simulink model "MRAC"  (R2022a)
settings: Solver=FixedStepAuto  StartTime=0.0  StopTime=25.0  FixedStep=0.0001  RelTol=1e-3
libraries: cstblocks x5
settings Model: Creator=loryb  LastModifiedBy=loryb

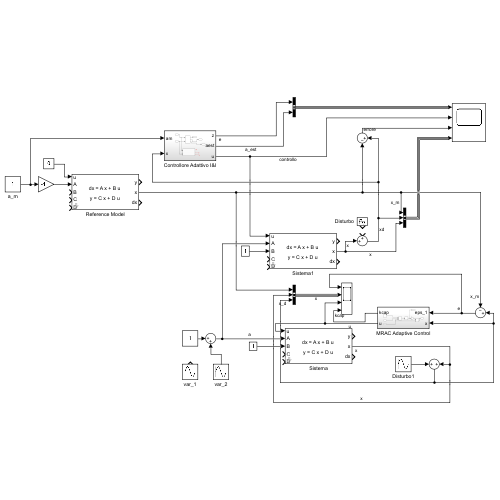
[thumbnail: Simulink's stored preview of the top-level diagram]
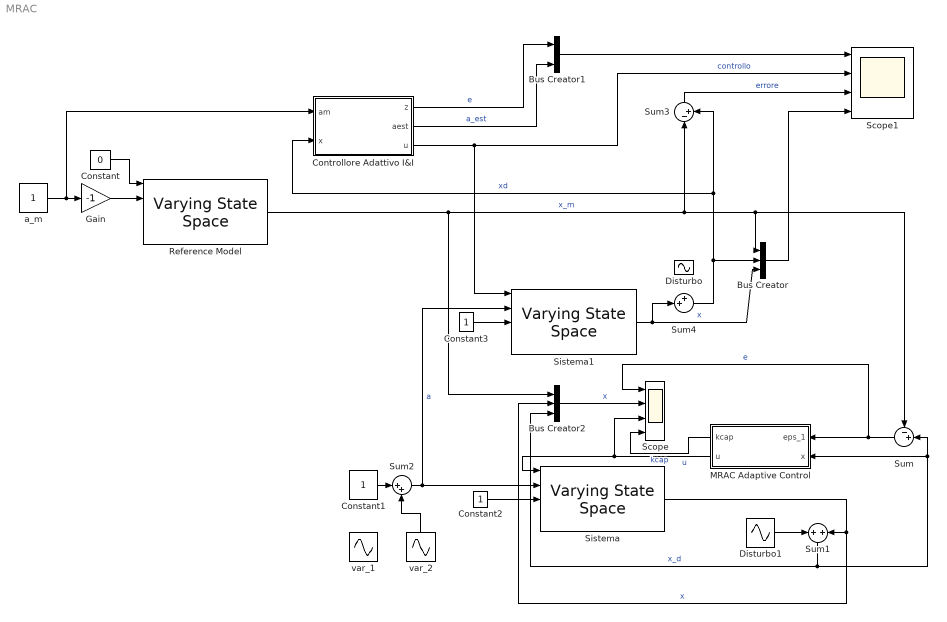
== system MRAC ==
  Bus Creator : BusCreator  Inputs=3
  Bus Creator1 : BusCreator  Inputs=2
  Bus Creator2 : BusCreator  Inputs=3
  Constant : Constant  Value=0
  Constant1 : Constant
  Constant2 : Constant
  Constant3 : Constant
  Controllore Adattivo I&I : Subsystem
  Disturbo : Sin  Amplitude=0.1  Frequency=1/5  SampleTime=0
  Disturbo1 : Sin  Amplitude=0.1  Frequency=1/5  SampleTime=0
  Gain : Gain  Gain=-1
  MRAC Adaptive Control : Subsystem
  Reference Model : cstblocks/Linear Parameter Varying/Varying State Space  x0=1  xNames=''  OutputX=on  OutputDX=on
  Scope : Scope  NumInputPorts=4
  Scope1 : Scope  NumInputPorts=4
  Sistema : cstblocks/Linear Parameter Varying/Varying State Space  x0=1  xNames=''  OutputX=on  OutputDX=on
  Sistema1 : cstblocks/Linear Parameter Varying/Varying State Space  x0=1  xNames=''  OutputX=on  OutputDX=on
  Sum : Sum  Inputs=-+|
  Sum1 : Sum  Inputs=+|+
  Sum2 : Sum  Inputs=|++
  Sum3 : Sum  Inputs=|-+
  Sum4 : Sum  Inputs=++|
  a_m : Constant
  var_1 : Sin  Amplitude=1/10  Frequency=10  SampleTime=0
  var_2 : Sin  Amplitude=10  Frequency=1/10  SampleTime=0
  wires:
  Constant/1 -> Reference Model/1
  Sum3/1 -> Scope1/3  "errore"
  Bus Creator/1 -> Scope1/4
  Controllore Adattivo I&I/1(z) -> Bus Creator1/1  "e"
  Sistema/2 -> Bus Creator2/2, Sum1/2  "x"
  Constant1/1 -> Sum2/1
  Constant3/1 -> Sistema1/3
  Bus Creator1/1 -> Scope1/1
  MRAC Adaptive Control/1(kcap) -> Scope/4  "kcap"
  Bus Creator2/1 -> Scope/2  "x"
  Constant2/1 -> Sistema/3
  Sum4/1 -> Bus Creator/2, Sum3/2, Controllore Adattivo I&I/2(x)  "xd"
  Sistema1/2 -> Bus Creator/3, Sum4/2  "x"
  Controllore Adattivo I&I/3(u) -> Scope1/2, Sistema1/1  "controllo"
  Sum2/1 -> Sistema1/2, Sistema/2  "a"
  Sum1/1 -> Bus Creator2/3, MRAC Adaptive Control/2(x), Sum/2  "x_d"
  MRAC Adaptive Control/2(u) -> Scope/3, Sistema/1  "u"
  Sum/1 -> Scope/1, MRAC Adaptive Control/1(eps_1)  "e"
  a_m/1 -> Gain/1, Controllore Adattivo I&I/1(am)
  Reference Model/2 -> Bus Creator/1, Sum/1, Sum3/1, Bus Creator2/1  "x_m"
  Controllore Adattivo I&I/2(aest) -> Bus Creator1/2  "a_est"
  Gain/1 -> Reference Model/2
  Disturbo1/1 -> Sum1/1
  var_2/1 -> Sum2/2

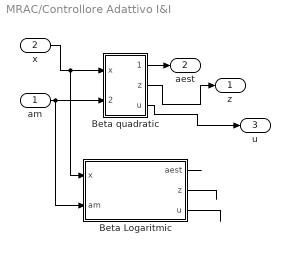
== system MRAC/Controllore Adattivo I&I ==
  am : Inport
  x : Inport  Port=2
  Beta Logaritmic : Subsystem
  Beta quadratic : Subsystem
  z : Outport
  aest : Outport  Port=2
  u : Outport  Port=3
  wires:
  x/1 -> Beta Logaritmic/1(x), Beta quadratic/1(x)
  am/1 -> Beta Logaritmic/2(am), Beta quadratic/2(am)
  Beta Logaritmic/1(aest) -> ?
  Beta Logaritmic/3(u) -> ?
  Beta Logaritmic/2(z) -> ?
  Beta quadratic/1(aest) -> aest/1
  Beta quadratic/2(z) -> z/1
  Beta quadratic/3(u) -> u/1

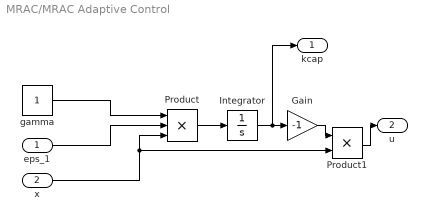
== system MRAC/MRAC Adaptive Control ==
  eps_1 : Inport
  x : Inport  Port=2
  Gain : Gain  Gain=-1
  Integrator : Integrator
  Product : Product  Inputs=3
  Product1 : Product
  gamma : Constant
  kcap : Outport
  u : Outport  Port=2
  wires:
  gamma/1 -> Product/1
  eps_1/1 -> Product/2
  x/1 -> Product/3, Product1/2
  Product/1 -> Integrator/1
  Integrator/1 -> kcap/1, Gain/1
  Gain/1 -> Product1/1
  Product1/1 -> u/1

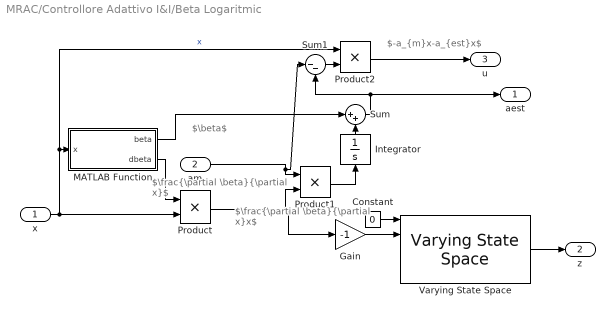
== system MRAC/Controllore Adattivo I&I/Beta Logaritmic ==
  note: $\frac{\partial \beta}{\partial x}$
  note: $\beta$
  note: $\frac{\partial \beta}{\partial x}x$
  note: $-a_{m}x-a_{est}x$
  x : Inport
  am : Inport  Port=2
  Constant : Constant  Value=0
  Gain : Gain  Gain=-1
  Integrator : Integrator
  MATLAB Function : MATLAB Function  TreatAsAtomicUnit=on
  Product : Product
  Product1 : Product
  Product2 : Product
  Sum : Sum  Inputs=|++
  Sum1 : Sum  Inputs=|--
  Varying State Space : cstblocks/Linear Parameter Varying/Varying State Space  x0=1  xNames=''  OutputX=on  OutputDX=on
  aest : Outport
  z : Outport  Port=2
  u : Outport  Port=3
  wires:
  x/1 -> Product/2, Product2/1, MATLAB Function/1(x)  "x"
  MATLAB Function/1(beta) -> Sum/1
  Sum/1 -> Sum1/2, aest/1
  Product/1 -> Gain/1, Product1/2
  MATLAB Function/2(dbeta) -> Product/1
  Gain/1 -> Varying State Space/2
  Varying State Space/2 -> z/1
  Constant/1 -> Varying State Space/1
  Sum1/1 -> Product2/2
  Product2/1 -> u/1
  Integrator/1 -> Sum/2
  Product1/1 -> Integrator/1
  am/1 -> Sum1/1, Product1/1

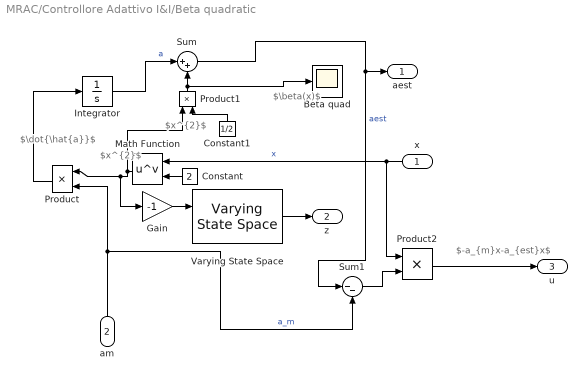
== system MRAC/Controllore Adattivo I&I/Beta quadratic ==
  note: $\beta(x)$
  note: $\dot{\hat{a}}$
  note: $x^{2}$
  note: $-a_{m}x-a_{est}x$
  note: $x^{2}$
  x : Inport
  am : Inport  Port=2
  Beta quad : Scope
  Constant : Constant  Value=2
  Constant1 : Constant  Value=1/2
  Gain : Gain  Gain=-1
  Integrator : Integrator
  Math Function : Math  Operator=pow
  Product : Product
  Product1 : Product
  Product2 : Product
  Sum : Sum  Inputs=|++
  Sum1 : Sum  Inputs=|--
  Varying State Space : cstblocks/Linear Parameter Varying/Varying State Space  x0=1  xNames=''  OutputX=on  OutputDX=on
  aest : Outport
  z : Outport  Port=2
  u : Outport  Port=3
  wires:
  Math Function/1 -> Product1/1, Gain/1, Product/1
  Constant/1 -> Math Function/2
  x/1 -> Product2/1, Math Function/1  "x"
  Product/1 -> Integrator/1
  Integrator/1 -> Sum/1  "a"
  Product1/1 -> Beta quad/1, Sum/2
  Constant1/1 -> Product1/2
  Sum/1 -> Sum1/1, aest/1  "aest"
  Gain/1 -> Varying State Space/2
  Varying State Space/2 -> z/1
  Product2/1 -> u/1
  Sum1/1 -> Product2/2
  am/1 -> Sum1/2, Product/2  "a_m"

== matlab function MRAC/Controllore Adattivo I&I/Beta Logaritmic/MATLAB Function ==
  data: x input; beta output; dbeta output
function [beta,dbeta] = betafun(x)
beta = 1/2*log(1+x^2);
dbeta=x/(1+x^2);
